simulink model "SIMULINK_anti0x2Dwindup_anti0x2Dsaturation"  (R2024b)
settings: Solver=ode45  StartTime=0.0  StopTime=1000  RelTol=1e-7  EnableMultiTasking=on
values from neighbouring files (symbols this model uses):
  gp_1 = gp_1/Gain_tec    [auto_ident_for_app.m]    (also in auto_ident_for_app_v2.m = identify(y1, u, t, 1, 0, true, NaN); auto_identification.m = gp_1 / Gain_tec)
  gp_2 = identify(y2, y1, t, 1, 0, true, 5)    [auto_ident_for_app.m]    (also in auto_ident_for_app_v2.m = identify(y2, y1, t, 1, 0, true, NaN))
  gp_3 = identify(y3, y2, t, 1, 0, false, 15)    [auto_ident_for_app.m]    (also in auto_ident_for_app_v2.m = evalin('base', 'gp_3'))
  Td = C.Kd / Kc    [actually_calculates_PID.m]
  Tf = C.Tf    [actually_calculates_PID.m]
  Ti = Kc / C.Ki    [actually_calculates_PID.m]
undefined symbols (not defined in the file or in its folder): kc, TEC
settings Model: Creator=LiberT  LastModifiedBy=Mathieu
settings SolverCC: AlgebraicLoopSolver=TrustRegion
settings DataIOCC: LimitDataPoints=on  SaveFormat=Array  SignalLoggingSaveFormat=ModelDataLogs  ReturnWorkspaceOutputs=off
settings OptimizationCC: BlockReduction=off  BooleanDataType=off  ExpressionDepthLimit=2147483647  InitFltsAndDblsToZero=on  LifeSpan=inf
settings DebuggingCC: SaveWithParameterizedLinksMsg=none  UnderspecifiedInitializationDetection=Classic  MergeDetectMultiDrivingBlocksExec=none  SignalResolutionControl=TryResolveAllWithWarning  MultiTaskDSMMsg=warning  MultiTaskCondExecSysMsg=none  FcnCallInpInsideContextMsg=warning  UnconnectedInputMsg=warning  UnconnectedOutputMsg=warning  UnconnectedLineMsg=warning  StateNameClashWarn=warning  SFUnexpectedBacktrackingDiag=warning  SFNoUnconditionalDefaultTransitionDiag=warning  SFExecutionAtInitializationDiag=none  ArithmeticOperatorsInVariantConditions=warning
settings HardwareCC: ProdBitPerPointer=32  ProdBitPerSizeT=32  ProdBitPerPtrDiffT=32  ProdLargestAtomicFloat=None  ProdIntDivRoundTo=Undefined  ProdEndianess=Unspecified  ProdWordSize=32  ProdHWDeviceType=32-bit Generic  TargetUnknown=on
settings ModelReferenceCC: EnableRefExpFcnMdlSchedulingChecks=on  PropagateSignalLabelsOutOfModel=off
settings SFSimCC: SimUseLocalCustomCode=off  CustomCodeUndefinedFunction=UseInterfaceOnly
settings RTWCC: RTWUseLocalCustomCode=off  GPUComputeCapability=3.5
settings CodeAppCC: StateflowObjectComments=on
settings GRTTargetCC: TargetFcnLib=ansi_tfl_tmw.mat  TargetLangStandard=C89/C90 (ANSI)  ModelReferenceCompliant=off  CompOptLevelCompliant=off  CombineOutputUpdateFcns=off  MatFileLogging=off  GRTInterface=on
settings ConfigComp: CovMetricSettings=dw  CovSaveCumulativeToWorkspaceVar=on  CovSaveSingleToWorkspaceVar=on  CovExternalEMLEnable=off

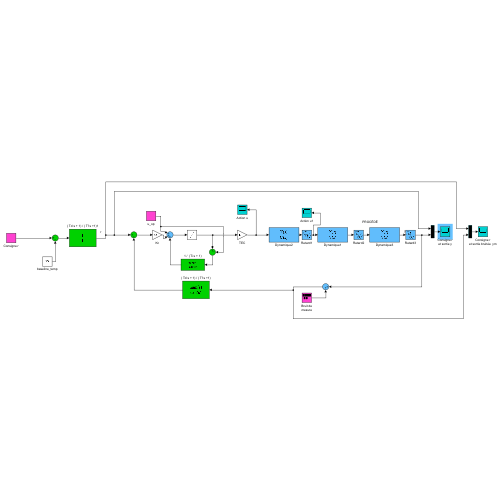
[thumbnail: Simulink's stored preview of the top-level diagram]
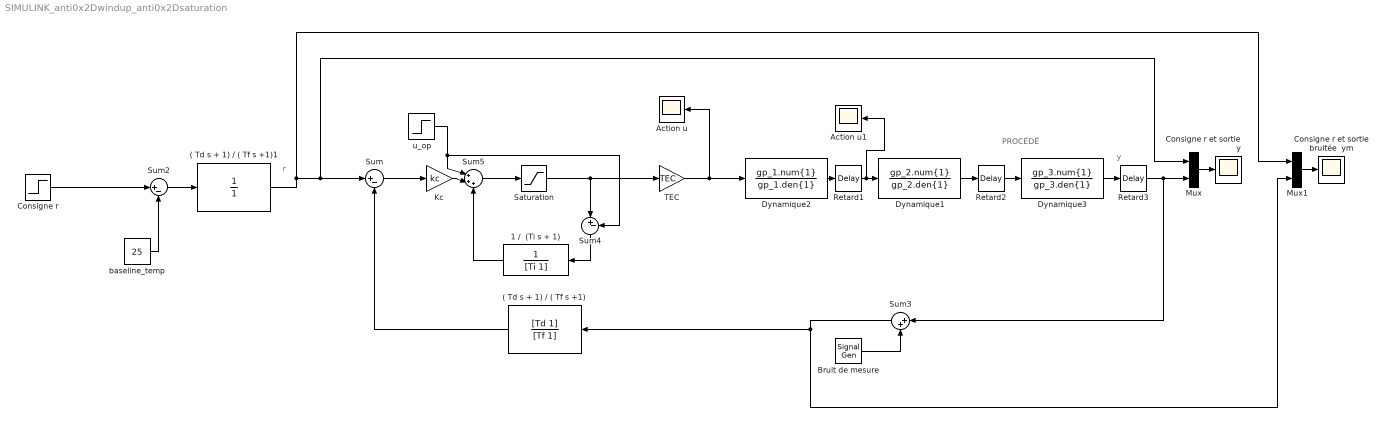
== system SIMULINK_anti0x2Dwindup_anti0x2Dsaturation ==
  note: PROCÉDÉ
  note: r
  note: y
  ( Td s + 1) / ( Tf s +1) : TransferFcn  Numerator=[Td 1]  Denominator=[Tf 1]
  ( Td s + 1) / ( Tf s +1)1 : TransferFcn  Denominator=[1]
  1 /  (Ti s + 1) : TransferFcn  Numerator=1  Denominator=[Ti 1]
  Action u : Scope
  Action u1 : Scope
  Bruit de mesure : SignalGenerator  Amplitude=0  Units=rad/sec
  Consigne r : Step  Time=1000  Before=30  After=30  SampleTime=0
  Consigne r et sortie bruitée  ym : Scope
  Consigne r et sortie y : Scope
  Dynamique1 : TransferFcn  Numerator=gp_2.num{1}  Denominator=gp_2.den{1}
  Dynamique2 : TransferFcn  Numerator=gp_1.num{1}  Denominator=gp_1.den{1}
  Dynamique3 : TransferFcn  Numerator=gp_3.num{1}  Denominator=gp_3.den{1}
  Kc : Gain  Gain=kc
  Mux : Mux  Inputs=2
  Mux1 : Mux  Inputs=2
  Retard1 : TransportDelay  DelayTime=gp_1.IODelay  BufferSize=5000
  Retard2 : TransportDelay  DelayTime=gp_2.IODelay  BufferSize=5000
  Retard3 : TransportDelay  DelayTime=gp_3.IODelay  BufferSize=5000
  Saturation : Saturate  UpperLimit=1  LowerLimit=-1
  Sum : Sum  Inputs=|+-  InputSameDT=on  SaturateOnIntegerOverflow=on  OutDataTypeStr=Inherit: Same as first input
  Sum2 : Sum  Inputs=|+-  InputSameDT=on  SaturateOnIntegerOverflow=on  OutDataTypeStr=Inherit: Same as first input
  Sum3 : Sum  Inputs=|++  InputSameDT=on  SaturateOnIntegerOverflow=on  OutDataTypeStr=Inherit: Same as first input
  Sum4 : Sum  Inputs=|+-  InputSameDT=on  SaturateOnIntegerOverflow=on  OutDataTypeStr=Inherit: Same as first input
  Sum5 : Sum  Inputs=|+++  InputSameDT=on  SaturateOnIntegerOverflow=on  OutDataTypeStr=Inherit: Same as first input
  TEC : Gain  Gain=TEC
  baseline_temp : Constant  Value=25
  u_op : Step  Time=50  Before=0.05  After=0.05  SampleTime=0
  wires:
  Saturation/1 -> TEC/1, Sum4/1
  Retard1/1 -> Action u1/1, Dynamique1/1
  Mux/1 -> Consigne r et sortie y/1
  Sum3/1 -> Mux1/2, ( Td s + 1) / ( Tf s +1)/1
  Bruit de mesure/1 -> Sum3/2
  Mux1/1 -> Consigne r et sortie bruitée  ym/1
  Dynamique2/1 -> Retard1/1
  u_op/1 -> Sum5/1, Sum4/2
  Sum4/1 -> 1 /  (Ti s + 1)/1
  1 /  (Ti s + 1)/1 -> Sum5/3
  Sum5/1 -> Saturation/1
  Kc/1 -> Sum5/2
  Sum/1 -> Kc/1
  ( Td s + 1) / ( Tf s +1)/1 -> Sum/2
  Consigne r/1 -> Sum2/1
  baseline_temp/1 -> Sum2/2
  Sum2/1 -> ( Td s + 1) / ( Tf s +1)1/1
  TEC/1 -> Dynamique2/1, Action u/1
  Dynamique1/1 -> Retard2/1
  Retard2/1 -> Dynamique3/1
  Dynamique3/1 -> Retard3/1
  Retard3/1 -> Mux/2, Sum3/1
  ( Td s + 1) / ( Tf s +1)1/1 -> Mux1/1, Sum/1, Mux/1
